simulink model "delay"  (R2024b)
settings: Solver=VariableStepAuto  StartTime=0.0  StopTime=10  RelTol=1e-3
undefined symbols (not defined in the file): dspblkCoreblockFVToolHelper, gcbh
settings Model: Creator=G5  LastModifiedBy=Administrator

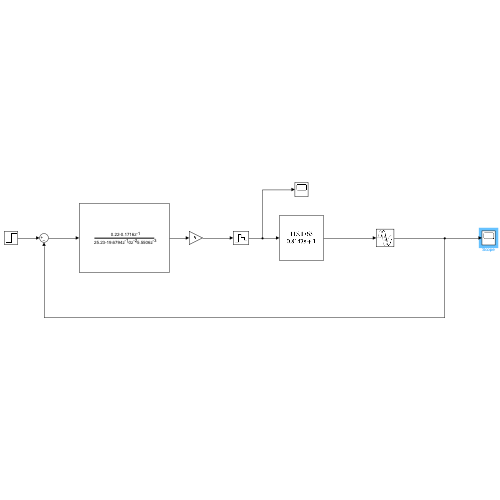
[thumbnail: Simulink's stored preview of the top-level diagram]
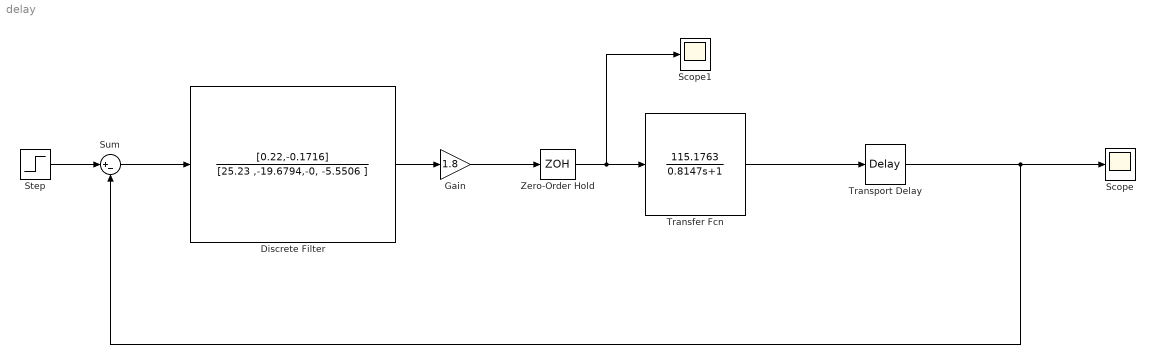
== system delay ==
  Discrete Filter : DiscreteFilter  LoadFcn=dspblkCoreblockFVToolHelper(gcbh,'load');  Numerator=[0.22,-0.1716]  Denominator=[25.23 ,-19.6794,-0, -5.5506 ]
      settings: CopyFcn=dspblkCoreblockFVToolHelper(gcbh,'copy');  DeleteFcn=dspblkCoreblockFVToolHelper(gcbh,'close');  ModelCloseFcn=dspblkCoreblockFVToolHelper(gcbh,'close');  PreSaveFcn=dspblkCoreblockFVToolHelper(gcbh,'presave');  PostSaveFcn=dspblkCoreblockFVToolHelper(gcbh,'postsave');  CloseFcn=dspblkCoreblockFVToolHelper(gcbh,'close');
  Gain : Gain  Gain=1.8
  Scope : Scope
  Scope1 : Scope
  Step : Step  SampleTime=0
  Sum : Sum  Inputs=|+-
  Transfer Fcn : TransferFcn  Numerator=[115.1763]  Denominator=[0.8147 1]
  Transport Delay : TransportDelay  DelayTime=0.4047
  Zero-Order Hold : ZeroOrderHold  SampleTime=0.20235
  wires:
  Step/1 -> Sum/1
  Transfer Fcn/1 -> Transport Delay/1
  Zero-Order Hold/1 -> Scope1/1, Transfer Fcn/1
  Sum/1 -> Discrete Filter/1
  Discrete Filter/1 -> Gain/1
  Gain/1 -> Zero-Order Hold/1
  Transport Delay/1 -> Sum/2, Scope/1
